simulink model "TwoLinkCartesianNN"  (Simulink 7.6)
settings: Solver=ode45  StartTime=0.0  StopTime=10.0  RelTol=1e-3
libraries: neural x148, roblocks x3, simulink x1
(part 1 of 5)
settings Model: Creator=mahyar  LastModifiedBy=mahyar

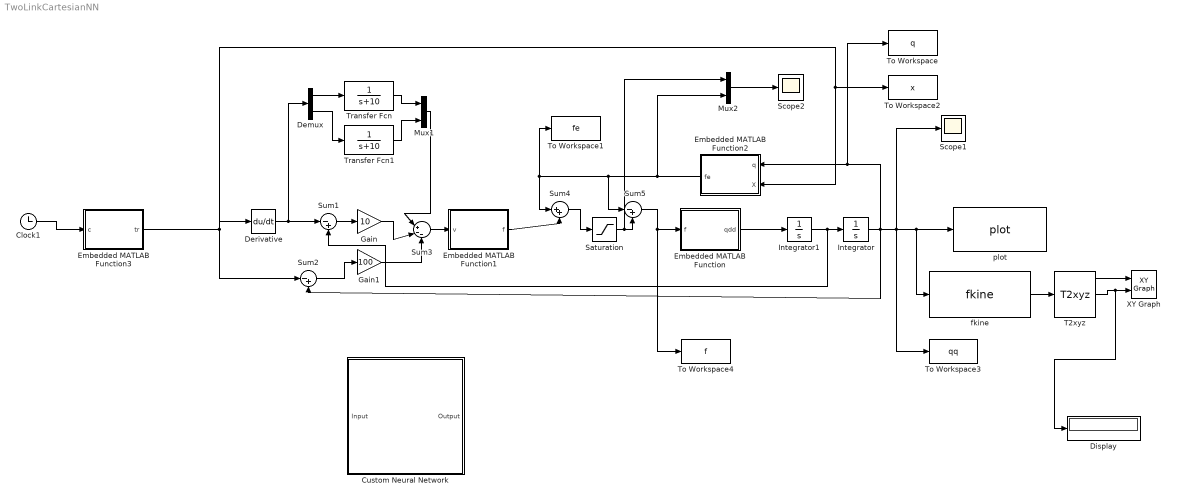
== system TwoLinkCartesianNN ==
  Clock1 : Clock
      settings: Decimation=10
  Custom Neural Network : Subsystem
      mask Description: Custom Neural Network
      mask Display: e = 0.06;c1 = [120 150 230]/255;c2 = ([120 150 230]+0)/383;c3 = ([120 150 230]+128)/383;patch([0 1 1 0],[0 0 1 1],c1);patch([0 1 1 1-e 1-e 0+e],[0 0 1 1-e 0+e 0+e],c2);patch([0 0 1 1-e 0+e 0+e],[0 1 1 1-e 1-e 0+e],c3);plot([0 1 1 0 0],[0 0 1 1 0]);fprintf('NNET');port_label('input',1,' Input');port_label('output',1,'Output ');
  Demux : Demux  Outputs=2
  Derivative : Derivative
  Display : Display
  Embedded MATLAB Function : Stateflow chart  TreatAsAtomicUnit=on
  Embedded MATLAB Function1 : Stateflow chart  TreatAsAtomicUnit=on
  Embedded MATLAB Function2 : Stateflow chart  TreatAsAtomicUnit=on
  Embedded MATLAB Function3 : Stateflow chart  TreatAsAtomicUnit=on
  Gain : Gain  Gain=10
  Gain1 : Gain  Gain=100
  Integrator : Integrator  InitialCondition=[0;0]
  Integrator1 : Integrator  InitialCondition=[0 ;0]
  Mux1 : Mux  Inputs=2
  Mux2 : Mux  Inputs=2
  Saturation : Saturate  UpperLimit=80  LowerLimit=-80
  Scope1 : Scope
      settings: YMin=0  YMax=1.2
  Scope2 : Scope
      settings: TimeRange=10  YMin=-7e+07  YMax=8e+07  SaveName=ScopeData2
  Sum1 : Sum  Inputs=|-+
  Sum2 : Sum  Inputs=|-+
  Sum3 : Sum  Inputs=|+--
  Sum4 : Sum  Inputs=|++
  Sum5 : Sum  Inputs=|-+
  T2xyz : roblocks/T2xyz  SystemSampleTime=-1
  To Workspace : ToWorkspace  VariableName=q  SampleTime=-1  SaveFormat=Structure
  To Workspace1 : ToWorkspace  VariableName=fe  SampleTime=-1  SaveFormat=Structure
  To Workspace2 : ToWorkspace  VariableName=x  SampleTime=-1  SaveFormat=Structure
  To Workspace3 : ToWorkspace  VariableName=qq  SampleTime=-1  SaveFormat=Structure
  To Workspace4 : ToWorkspace  VariableName=f  SampleTime=-1  SaveFormat=Structure
  Transfer Fcn : TransferFcn  Denominator=[1 10]
  Transfer Fcn1 : TransferFcn  Denominator=[1 10]
  XY Graph : simulink/Sinks/XY Graph  SystemSampleTime=-1  xmin=-4  xmax=4  ymin=-4  ymax=4  st=-1
  fkine : roblocks/fkine  SystemSampleTime=-1  robot=r
  plot : roblocks/plot  SystemSampleTime=-1  robot=r
  wires:
  fkine/1 -> T2xyz/1
  Embedded MATLAB Function/1(qdd) -> Integrator1/1
  Integrator/1 -> plot/1, fkine/1, Scope1/1, To Workspace3/1, Sum2/2, Embedded MATLAB Function2/1(q), To Workspace/1
  Integrator1/1 -> Integrator/1, Sum1/2
  Derivative/1 -> Sum1/1, Demux/1
  Sum3/1 -> Embedded MATLAB Function1/1(v)
  Sum1/1 -> Gain/1
  Gain/1 -> Sum3/2
  Sum2/1 -> Gain1/1
  Gain1/1 -> Sum3/3
  Demux/1 -> Transfer Fcn/1
  Demux/2 -> Transfer Fcn1/1
  Transfer Fcn/1 -> Mux1/1
  Transfer Fcn1/1 -> Mux1/2
  Mux1/1 -> Sum3/1
  Embedded MATLAB Function2/1(fe) -> Mux2/2, Sum5/1, Sum4/1, To Workspace1/1
  Mux2/1 -> Scope2/1
  Embedded MATLAB Function1/1(f) -> Sum4/2
  Embedded MATLAB Function3/1(tr) -> Derivative/1, Sum2/1, Embedded MATLAB Function2/2(X), To Workspace2/1
  T2xyz/1 -> XY Graph/1
  T2xyz/2 -> XY Graph/2, Display/1
  Sum5/1 -> Embedded MATLAB Function/1(f), To Workspace4/1
  Sum4/1 -> Saturation/1
  Saturation/1 -> Sum5/2, Mux2/1
  Clock1/1 -> Embedded MATLAB Function3/1(c)

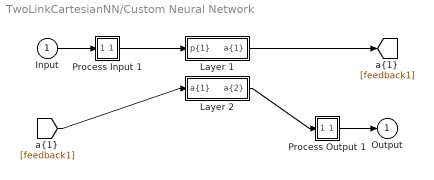
== system TwoLinkCartesianNN/Custom Neural Network ==
  Input : Inport  PortDimensions=131
      mask Display: e = 0.06;c1 = [120 230 180]/255;c2 = ([120 230 180]+0)/(256+128);c3 = ([120 230 180]+128)/(256+128);patch([0 1 1 0],[0 0 1 1],c1);patch([0 1 1 1-e 1-e 0+e],[0 0 1 1-e 0+e 0+e],c2);patch([0 0 1 1-e 0+e 0+e],[0 1 1 1-e 1-e 0+e],c3);plot([0 1 1 0 0],[0 0 1 1 0]);
  Layer 1 : Subsystem
      mask Display: e = 0.06;c1 = [120 150 230]/255;c2 = ([120 150 230]+0)/383;c3 = ([120 150 230]+128)/383;patch([0 1 1 0],[0 0 1 1],c1);patch([0 1 1 1-e 1-e 0+e],[0 0 1 1-e 0+e 0+e],c2);patch([0 0 1 1-e 0+e 0+e],[0 1 1 1-e 1-e 0+e],c3);plot([0 1 1 0 0],[0 0 1 1 0]);
  Layer 2 : Subsystem
      mask Display: e = 0.06;c1 = [120 150 230]/255;c2 = ([120 150 230]+0)/383;c3 = ([120 150 230]+128)/383;patch([0 1 1 0],[0 0 1 1],c1);patch([0 1 1 1-e 1-e 0+e],[0 0 1 1-e 0+e 0+e],c2);patch([0 0 1 1-e 0+e 0+e],[0 1 1 1-e 1-e 0+e],c3);plot([0 1 1 0 0],[0 0 1 1 0]);
  Process Input 1 : Subsystem
      mask Display: e = 0.06;c1 = [120 150 230]/255;c2 = ([120 150 230]+0)/383;c3 = ([120 150 230]+128)/383;patch([0 1 1 0],[0 0 1 1],c1);patch([0 1 1 1-e 1-e 0+e],[0 0 1 1-e 0+e 0+e],c2);patch([0 0 1 1-e 0+e 0+e],[0 1 1 1-e 1-e 0+e],c3);plot([0 1 1 0 0],[0 0 1 1 0]);
  Process Output 1 : Subsystem
      mask Display: e = 0.06;c1 = [120 150 230]/255;c2 = ([120 150 230]+0)/383;c3 = ([120 150 230]+128)/383;patch([0 1 1 0],[0 0 1 1],c1);patch([0 1 1 1-e 1-e 0+e],[0 0 1 1-e 0+e 0+e],c2);patch([0 0 1 1-e 0+e 0+e],[0 1 1 1-e 1-e 0+e],c3);plot([0 1 1 0 0],[0 0 1 1 0]);
  Output : Outport  InitialOutput=[0;0;0;0;0;0;0;0;0;0;0;0;0;0;0;0;0;0;0;0;0;0;0;0;0;0;0;0;0;0;0;0;0;0;0;0;0;0;0;0;0;0;0;0;0;0;0;0;0;0;0;0;0;0;0;0;0;0;0;0;0;0;0;0;0;0;0;0;0;0;0;0;0;0;0;0;0;0;0;0;0;0;0;0;0;0;0;0;0;0;0;0;0;0;0;0;0;0;0;0;0;0;0;0;0;0;0;0;0;0;0;0;0;0;0;0;0;0;0;0;0;0;0;0;0;0;0;0;0;0;0]
      mask Display: e = 0.06;c1 = [120 230 180]/255;c2 = ([120 230 180]+0)/(256+128);c3 = ([120 230 180]+128)/(256+128);patch([0 1 1 0],[0 0 1 1],c1);patch([0 1 1 1-e 1-e 0+e],[0 0 1 1-e 0+e 0+e],c2);patch([0 0 1 1-e 0+e 0+e],[0 1 1 1-e 1-e 0+e],c3);plot([0 1 1 0 0],[0 0 1 1 0]);
  wires:
  Input/1 -> Process Input 1/1(x)
  Process Output 1/1(y) -> Output/1
  Process Input 1/1(p) -> Layer 1/1("p{1}")
  Layer 1/1("a{1}") -> [feedback1]
  [feedback1] -> Layer 2/1("a{1} ")
  Layer 2/1("a{2}") -> Process Output 1/1(a)

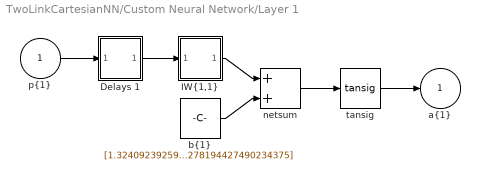
== system TwoLinkCartesianNN/Custom Neural Network/Layer 1 ==
  "p{1}" : Inport  PortDimensions=130
      mask Display: e = 0.06;c1 = [120 230 180]/255;c2 = ([120 230 180]+0)/(256+128);c3 = ([120 230 180]+128)/(256+128);patch([0 1 1 0],[0 0 1 1],c1);patch([0 1 1 1-e 1-e 0+e],[0 0 1 1-e 0+e 0+e],c2);patch([0 0 1 1-e 0+e 0+e],[0 1 1 1-e 1-e 0+e],c3);plot([0 1 1 0 0],[0 0 1 1 0]);
  Delays 1 : Subsystem
      mask Display: e = 0.06;c1 = [120 150 230]/255;c2 = ([120 150 230]+0)/383;c3 = ([120 150 230]+128)/383;patch([0 1 1 0],[0 0 1 1],c1);patch([0 1 1 1-e 1-e 0+e],[0 0 1 1-e 0+e 0+e],c2);patch([0 0 1 1-e 0+e 0+e],[0 1 1 1-e 1-e 0+e],c3);plot([0 1 1 0 0],[0 0 1 1 0]);disp('0');
  "IW{1,1}" : Subsystem
      mask Display: e = 0.06;c1 = [120 150 230]/255;c2 = ([120 150 230]+0)/383;c3 = ([120 150 230]+128)/383;patch([0 1 1 0],[0 0 1 1],c1);patch([0 1 1 1-e 1-e 0+e],[0 0 1 1-e 0+e 0+e],c2);patch([0 0 1 1-e 0+e 0+e],[0 1 1 1-e 1-e 0+e],c3);plot([0 1 1 0 0],[0 0 1 1 0]);disp('W');
  "b{1}" : Constant  Value=[1.3240923925958092421950595962698571383953094482421875;-0.5504773511715745915040542968199588358402252197265625;0.6676637199418795631800094270147383213043212890625;-1.0007797988375102260505400408874265849590301513671875;0.00220576829502830938645185909763313247822225093841552734375;-0.86926988321640508150522919095237739384174346923828125;-0.37316467032025213423906961907050572335720062255859375;-0.99766857705958400526213836201350204646587371826171875;-0.8715553818086945181420333028654567897319793701171875;-1.9230157011015316381730144712491892278194427490234375]
      mask Display: e = 0.06;c1 = [120 150 230]/255;c2 = ([120 150 230]+0)/383;c3 = ([120 150 230]+128)/383;patch([0 1 1 0],[0 0 1 1],c1);patch([0 1 1 1-e 1-e 0+e],[0 0 1 1-e 0+e 0+e],c2);patch([0 0 1 1-e 0+e 0+e],[0 1 1 1-e 1-e 0+e],c3);plot([0 1 1 0 0],[0 0 1 1 0]);disp('b');
  netsum : Sum  Inputs=2  SaturateOnIntegerOverflow=on  InputSameDT=on  OutDataTypeStr=Inherit: Same as first input
      mask Display: e = 0.06;c1 = [120 150 230]/255;c2 = ([120 150 230]+0)/383;c3 = ([120 150 230]+128)/383;patch([0 1 1 0],[0 0 1 1],c1);patch([0 1 1 1-e 1-e 0+e],[0 0 1 1-e 0+e 0+e],c2);patch([0 0 1 1-e 0+e 0+e],[0 1 1 1-e 1-e 0+e],c3);plot([0 1 1 0 0],[0 0 1 1 0]);disp('+');
  tansig : neural/Transfer Functions/tansig  SystemSampleTime=-1
  "a{1}" : Outport  InitialOutput=[0;0;0;0;0;0;0;0;0;0]
      mask Display: e = 0.06;c1 = [120 230 180]/255;c2 = ([120 230 180]+0)/(256+128);c3 = ([120 230 180]+128)/(256+128);patch([0 1 1 0],[0 0 1 1],c1);patch([0 1 1 1-e 1-e 0+e],[0 0 1 1-e 0+e 0+e],c2);patch([0 0 1 1-e 0+e 0+e],[0 1 1 1-e 1-e 0+e],c3);plot([0 1 1 0 0],[0 0 1 1 0]);
  wires:
  "p{1}"/1 -> Delays 1/1("p{1}")
  Delays 1/1("pd{1,1}") -> "IW{1,1}"/1("pd{1,1}")
  "IW{1,1}"/1("iz{1,1}") -> netsum/1
  "b{1}"/1 -> netsum/2
  netsum/1 -> tansig/1
  tansig/1 -> "a{1}"/1

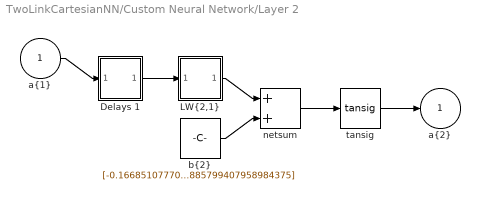
== system TwoLinkCartesianNN/Custom Neural Network/Layer 2 ==
  "a{1} " : Inport  PortDimensions=10
      mask Display: e = 0.06;c1 = [120 230 180]/255;c2 = ([120 230 180]+0)/(256+128);c3 = ([120 230 180]+128)/(256+128);patch([0 1 1 0],[0 0 1 1],c1);patch([0 1 1 1-e 1-e 0+e],[0 0 1 1-e 0+e 0+e],c2);patch([0 0 1 1-e 0+e 0+e],[0 1 1 1-e 1-e 0+e],c3);plot([0 1 1 0 0],[0 0 1 1 0]);
  Delays 1 : Subsystem
      mask Display: e = 0.06;c1 = [120 150 230]/255;c2 = ([120 150 230]+0)/383;c3 = ([120 150 230]+128)/383;patch([0 1 1 0],[0 0 1 1],c1);patch([0 1 1 1-e 1-e 0+e],[0 0 1 1-e 0+e 0+e],c2);patch([0 0 1 1-e 0+e 0+e],[0 1 1 1-e 1-e 0+e],c3);plot([0 1 1 0 0],[0 0 1 1 0]);disp('0');
  "LW{2,1}" : Subsystem
      mask Display: e = 0.06;c1 = [120 150 230]/255;c2 = ([120 150 230]+0)/383;c3 = ([120 150 230]+128)/383;patch([0 1 1 0],[0 0 1 1],c1);patch([0 1 1 1-e 1-e 0+e],[0 0 1 1-e 0+e 0+e],c2);patch([0 0 1 1-e 0+e 0+e],[0 1 1 1-e 1-e 0+e],c3);plot([0 1 1 0 0],[0 0 1 1 0]);disp('W');
  "b{2}" : Constant  Value=[-0.166851077700779837353906032149097882211208343505859375;-0.7843861402824192641247691426542587578296661376953125;-1.21899199102033239938691622228361666202545166015625;0.74462505282958513230795460913213901221752166748046875;-14.41248836651606524128510500304400920867919921875;-0.50346793045477788997033030682359822094440460205078125;-0.08879336411781564575296243901902926154434680938720703125;0.5949153939878153440901087378733791410923004150390625;-0.23842351826200747222372910982812754809856414794921875;0.08428080431664590477236487231493811123073101043701171875;2.475390507348269597542866904404945671558380126953125;-1.515487985379832647225839536986313760280609130859375;-1.4841112529706073086543938188697211444377899169921875;-3.698697968380269873733823260408826172351837158203125;1.3190452876237037660445139408693648874759674072265625;-0.577684328874242591922438805340789258480072021484375;0.37709011321786067849615164959686808288097381591796875;4.10059286012625623385474682436324656009674072265625;-1.32830989378755948138177700457163155078887939453125;-0.640354700549860211822306155227124691009521484375;-0.9377771361900177904402653439319692552089691162109375;-0.332323286094457659434198149028816260397434234619140625;-0.491597104001876006318383360849111340939998626708984375;-0.33628881344515093587688170373439788818359375;-0.89967439422496031653508907766081392765045166015625;-0.6323618525322995953530380575102753937244415283203125;0.68337225464510320538380483412765897810459136962890625;0.2793558622674485736325777907040901482105255126953125;-0.201525497936521802433418315558810718357563018798828125;0.11879681172828326918278207813273184001445770263671875;-0.00629195051082419298804637719513266347348690032958984375;0.315698408201655678073649369252962060272693634033203125;0.2548898739333729235312375749344937503337860107421875;-0.94370324940252425793829615940921939909458160400390625;-0.47721574682566070269018609906197525560855865478515625;-0.41159665142540247106950346278608776628971099853515625;-0.59614215420473015694113883000682108104228973388671875;-0.45437374897230331516340129383024759590625762939453125;0.325243631150170298127477508387528359889984130859375;0.020432118758119656443117406752207898534834384918212890625;-0.0738731793699264616126498594894655980169773101806640625;-0.14508218113239390589797039865516126155853271484375;0.1505264641359329302883196533002774231135845184326171875;-0.06821648328257075288849620164910447783768177032470703125;-0.231870568506500174255080537477624602615833282470703125;0.0967403775629794016044371574025717563927173614501953125;0.57078388551450431886991054852842353284358978271484375;1.045708075089812449931514493073336780071258544921875;1.3787610353289398990028757907566614449024200439453125;0.339027955795436763963834891910664737224578857421875;0.545951479721761501195942400954663753509521484375;0.09048094402358418386622673779129399918019771575927734375;-0.812040329819399442357052976149134337902069091796875;-0.0553867262122519632416839385768980719149112701416015625;-0.66903156004904129616761565557681024074554443359375;-0.1815240657789118638998360211189719848334789276123046875;-0.6668235261192074769809323697700165212154388427734375;-0.35750263343022792295045064747682772576808929443359375;0.0827722526877872066819463725551031529903411865234375;0.251478809341716014191803196808905340731143951416015625;4.52587391069360034379087665001861751079559326171875;-0.05396634953846461690840641267641331069171428680419921875;0.01061590559154333701652461741105071268975734710693359375;0.50455607095879084766920641413889825344085693359375;-0.0661537821694408723072200473325210623443126678466796875;0.0205873683818567389247622401171611272729933261871337890625;-0.1439892528579400643451435826136730611324310302734375;0.28208297214947375408655716455541551113128662109375;0.11076787990505952696818070535300648771226406097412109375;-0.467520686277630714844377735062153078615665435791015625;0.0564319078922222161498467585261096246540546417236328125 ...(+3348 chars)]
      mask Display: e = 0.06;c1 = [120 150 230]/255;c2 = ([120 150 230]+0)/383;c3 = ([120 150 230]+128)/383;patch([0 1 1 0],[0 0 1 1],c1);patch([0 1 1 1-e 1-e 0+e],[0 0 1 1-e 0+e 0+e],c2);patch([0 0 1 1-e 0+e 0+e],[0 1 1 1-e 1-e 0+e],c3);plot([0 1 1 0 0],[0 0 1 1 0]);disp('b');
  netsum : Sum  Inputs=2  SaturateOnIntegerOverflow=on  InputSameDT=on  OutDataTypeStr=Inherit: Same as first input
      mask Display: e = 0.06;c1 = [120 150 230]/255;c2 = ([120 150 230]+0)/383;c3 = ([120 150 230]+128)/383;patch([0 1 1 0],[0 0 1 1],c1);patch([0 1 1 1-e 1-e 0+e],[0 0 1 1-e 0+e 0+e],c2);patch([0 0 1 1-e 0+e 0+e],[0 1 1 1-e 1-e 0+e],c3);plot([0 1 1 0 0],[0 0 1 1 0]);disp('+');
  tansig : neural/Transfer Functions/tansig  SystemSampleTime=-1
  "a{2}" : Outport  InitialOutput=[0;0;0;0;0;0;0;0;0;0;0;0;0;0;0;0;0;0;0;0;0;0;0;0;0;0;0;0;0;0;0;0;0;0;0;0;0;0;0;0;0;0;0;0;0;0;0;0;0;0;0;0;0;0;0;0;0;0;0;0;0;0;0;0;0;0;0;0;0;0;0;0;0;0;0;0;0;0;0;0;0;0;0;0;0;0;0;0;0;0;0;0;0;0;0;0;0;0;0;0;0;0;0;0;0;0;0;0;0;0;0;0;0;0;0;0;0;0;0;0;0;0;0;0;0;0;0;0;0;0;0]
      mask Display: e = 0.06;c1 = [120 230 180]/255;c2 = ([120 230 180]+0)/(256+128);c3 = ([120 230 180]+128)/(256+128);patch([0 1 1 0],[0 0 1 1],c1);patch([0 1 1 1-e 1-e 0+e],[0 0 1 1-e 0+e 0+e],c2);patch([0 0 1 1-e 0+e 0+e],[0 1 1 1-e 1-e 0+e],c3);plot([0 1 1 0 0],[0 0 1 1 0]);
  wires:
  "a{1} "/1 -> Delays 1/1("p{2}")
  Delays 1/1("pd{2,1}") -> "LW{2,1}"/1("ad{2,1}")
  "LW{2,1}"/1("lz{2,1}") -> netsum/1
  "b{2}"/1 -> netsum/2
  netsum/1 -> tansig/1
  tansig/1 -> "a{2}"/1

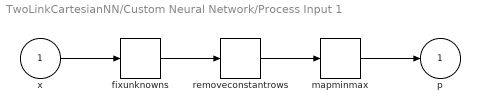
== system TwoLinkCartesianNN/Custom Neural Network/Process Input 1 ==
  x : Inport  PortDimensions=131
      mask Display: e = 0.06;c1 = [120 230 180]/255;c2 = ([120 230 180]+0)/(256+128);c3 = ([120 230 180]+128)/(256+128);patch([0 1 1 0],[0 0 1 1],c1);patch([0 1 1 1-e 1-e 0+e],[0 0 1 1-e 0+e 0+e],c2);patch([0 0 1 1-e 0+e 0+e],[0 1 1 1-e 1-e 0+e],c3);plot([0 1 1 0 0],[0 0 1 1 0]);
  fixunknowns : neural/Processing Functions/fixunknowns  SystemSampleTime=-1  inputSize=131  indices=[1 2 3 4 5 6 7 8 9 10 11 12 13 14 15 16 17 18 19 20 21 22 23 24 25 26 27 28 29 30 31 32 33 34 35 36 37 38 39 40 41 42 43 44 45 46 47 48 49 50 51 52 53 54 55 56 57 58 59 60 61 62 63 64 65 66 67 68 69 70 71 72 73 74 75 76 77 78 79 80 81 82 83 84 85 86 87 88 89 90 91 92 93 94 95 96 97 98 99 100 101 102 103 104 105 106 107 108 109 110 111 112 113 114 115 116 117 118 119 120 121 122 123 124 125 126 127 128 129 130 131]
  mapminmax : neural/Processing Functions/mapminmax  SystemSampleTime=-1  xmin=[0;0;0;0;0;0;0;0;0;0;0;0;0;0;0;0;0;0;0;0;0;0;0;0;0;0;0;0;0;0;0;0;0;0;0;0;0;0;0;0;0;0;0;0;0;0;0;0;0;0;0;0;0;0;0;0;0;0;0;0;0;0;0;0;0;0;0;0;0;0;0;0;3.39127133697992125941339678186e-14;1.94155593837782758925184781959e-13;3.54398474305817057411433895115e-13;5.14641354773887706608195592496e-13;8.35127115710133614268638535189e-13;1.47609863758305467089616051929e-12;2.75804168133061354742935714575e-12;5.32192776883259754581479408544e-12;1.04496999438640321394489766045e-11;2.07052442940367709453448439864e-11;4.12163329948217238004723203404e-11;8.22385103981495304840702394091e-11;1.64282865211836786518729156413e-10;3.28371574867337765860322736756e-10;6.56548994290845593632612882786e-10;1.31290383358788472553360511622e-09;2.62561351398205710155639048685e-09;5.25103288197077871607547111966e-09;1.05018716467497244319239966333e-08;2.10035492915136274652237297587e-08;4.20069050418654633946216733417e-08;8.40136183858650958859338596547e-08;1.68027052447046628446737127904e-07;3.36053950062127196587373305359e-07;6.72107863263064430166737403538e-07;1.34421616154729239181009163573e-06;2.68843464563915471185690311828e-06;5.37687916386845021879435993495e-06;1.07537984001248827033072469339e-05;2.15077576687536199326333807846e-05;4.30161593658708241898550039828e-05;8.6034895202718170820720133829e-05;0.000172080095072320640985780171306;0.00034420139499983192204329851549;0.000688567494861905748590458209435;0.00137779288890775087131346232638;0.00275821001284331027147977977165;0.00552685813998672961777636203351;0.0110949992805678375462630214088;0.0223513934671833273959418164623;0.0453187697715917506280369764227;0.0928695870897397468546330401296;0.192893077264244983126673105289;0.401559002740551396204438105997;0.550000000000000044408920985006;0.550000000000000044408920985006;0.550000000000000044408920985006;0.550000000000000044408920985006;0.550000000000000044408920985006;0.550000000000000044408920985006;0.550000000000000044408920985006;0.550000000000000044408920985006;0.550000000000000044408920985006;0.550000000000000044408920985006;0.550000000000000044408920985006;0.550000000000000044408920985006;0.550000000000000044408920985006;0.550000000000000044408920985006]  xmax=[6.68564073621395946207252206599e-10;2.40683066503702594401350610322e-08;6.42490074750161794335371646947e-07;1.62701752956502980549790410292e-05;0.000407798010910180759591714405587;0.0102001724267335759643859915968;0.0590865656757802448773020387307;0.05908656567578192408962678428;0.248304885285112464377021979089;0.448669105191036199364873482409;0.5890397005128985563615628962;0.637646357032778721141141886619;0.603709527915894494931592362263;0.557523021740516044886248891999;0.536800209363013203223147229437;0.540689393306072352274327386112;0.55058918842240767155260527943;0.552055136888254360805206033547;0.550032803944412118646312137571;0.549750172599031472486785787623;0.550009364327472938249741218897;0.550029657512358438609112454287;0.549997287887633579117618864984;0.549996564654723352205678565952;0.550000510600512027004072024283;0.550000387452318162395670242404;0.549999917700721319135936937528;0.549999957619495050131774860347;0.550000012194730936165854018327;0.550000004465412195564510966506;0.549999998289805169804367324105;0.549999999552185592222031118581;0.550000000230323027317069772835;0.550000000041772296732744962355;0.549999999969969621815835125744;0.549999999996559352233305162372;0.550000000003808553472595122003;0.550000000000212208028926852421;0.549999999999528976779572531086;0.549999999999999600319711134944;0.550000000000056887827781793021;0.549999999999997046806754497084;0.549999999999993383070773234067;0.550000000000000821565038222616;0.550000000000000821565038222616;0.549999999999999933386618522491;0.549999999999999933386618522491;0.550000000000000155431223447522;0.550000000000000155431223447522;0.550000000000000044408920985006;0.550000000000000044408920985006;0.550000000000000044408920985006;0.550000000000000044408920985006;0.550000000000000044408920985006;0.550000000000000044408920985006;0.550000000000000044408920985006;0.550000000000000044408920985006;0.550000000000000044408920985006;0.550000000000000044408920985006;0.550000000000000044408920985006;0.550000000000000044408920985006;0.550000000000000044408920985006;0.550000000000000044408920985006;0.550000000000000044408920985006;0.550000000000000044408920985006;0.550000000000000044408920985006;0.550000000000000044408920985006;0.550000000000000044408920985006;0.550000000000000044408920985006;0.550000000000000044408920985006;0.550000000000000044408920985006;0.550000000000000044408920985006;0.550000000000000044408920985006;0.550000000000000044408920985006;0.550000000000000044408920985006;0.550000000000000044408920985006;0.550000000000000044408920985006;0.550000000000000044408920985006;0.550000000000000044408920985006;0.550000000000000044408920985006;0.550000000000000044408920985006;0.550000000000000044408920985006;0.550000000000000044408920985006;0.550000000000000044408920985006;0.550000000000000044408920985006;0.550000000000000044408920985006;0.550000000000000044408920985006;0.550000000000000044408920985006;0.550000000000000044408920985006;0.550000000000000044408920985006;0.550000000000000044408920985006;0.550000000000000044408920985006;0.550000000000000044408920985006;0.550000000000000044408920985006;0.550000000000000044408920985006;0.550000000000000044408920985006;0.550000000000000044408920985006;0.550000000000000044408920985006;0.550000000000000044408920985006;0.550000000000000044408920985006;0.550000000000000044408920985006;0.550000000000000044408920985006;0.550000000000000044408920985006;0.550000000000000044408920985006;0.550000000000000044408920985006;0.550000000000000044408920985006;0.550000000000000044408920985006;0.550000000000000044408920985006;0.550000000000000044408920985006;0.550000000000000044408920985006;0.550000000000000044408920985006;0.550000000000000044408920985006;0.550000000000000044408920985006;0.550000000000000044408920985006;0.550000000000000044408920985006;0.550000000000000044408920985006;0.785743985268398059673700117855;1.10432497606786705901527056994;1.20164413042005158160918654175;1.12195081313582667448258689546;1.01691014230244780591760900279;0.969569261404452320540769960644;0.978680394311837176246626768261;1.00093087950283621267999478732;1.00483647144235255233013504039;1.00015124969759061634988484002;0.999408144611358295605896273628;1.00001331279962646370051970734;1.00007073431991133638518931548;1.00000940511901337259814681602]  ymin=-1  ymax=1
  removeconstantrows : neural/Processing Functions/removeconstantrows  SystemSampleTime=-1  inputSize=131  keep=[2 3 4 5 6 7 8 9 10 11 12 13 14 15 16 17 18 19 20 21 22 23 24 25 26 27 28 29 30 31 32 33 34 35 36 37 38 39 40 41 42 43 44 45 46 47 48 49 50 51 52 53 54 55 56 57 58 59 60 61 62 63 64 65 66 67 68 69 70 71 72 73 74 75 76 77 78 79 80 81 82 83 84 85 86 87 88 89 90 91 92 93 94 95 96 97 98 99 100 101 102 103 104 105 106 107 108 109 110 111 112 113 114 115 116 117 118 119 120 121 122 123 124 125 126 127 128 129 130 131]
  p : Outport  PortDimensions=130
      mask Display: e = 0.06;c1 = [120 230 180]/255;c2 = ([120 230 180]+0)/(256+128);c3 = ([120 230 180]+128)/(256+128);patch([0 1 1 0],[0 0 1 1],c1);patch([0 1 1 1-e 1-e 0+e],[0 0 1 1-e 0+e 0+e],c2);patch([0 0 1 1-e 0+e 0+e],[0 1 1 1-e 1-e 0+e],c3);plot([0 1 1 0 0],[0 0 1 1 0]);
  wires:
  x/1 -> fixunknowns/1
  fixunknowns/1 -> removeconstantrows/1
  removeconstantrows/1 -> mapminmax/1
  mapminmax/1 -> p/1

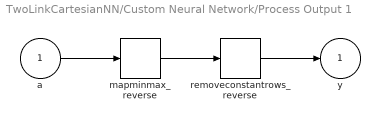
== system TwoLinkCartesianNN/Custom Neural Network/Process Output 1 ==
  a : Inport  PortDimensions=131
      mask Display: e = 0.06;c1 = [120 230 180]/255;c2 = ([120 230 180]+0)/(256+128);c3 = ([120 230 180]+128)/(256+128);patch([0 1 1 0],[0 0 1 1],c1);patch([0 1 1 1-e 1-e 0+e],[0 0 1 1-e 0+e 0+e],c2);patch([0 0 1 1-e 0+e 0+e],[0 1 1 1-e 1-e 0+e],c3);plot([0 1 1 0 0],[0 0 1 1 0]);
  mapminmax_reverse : neural/Processing Functions/mapminmax_reverse  SystemSampleTime=-1  xmin=[0;0;0;0;0;0;0;0;0;0;-7.69111613108554337259192834608;-11.3245418689005283852111460874;0;0;0;0;0;0;0;0;0;0;0;0;0;0;0;0;0;0;0;0;0;0;0;0;0;0;0;0;0;0;0;0;0;0;0;0;0;0;0;0;0;0;0;0;0;0;0;0;0;0;0;0;0;0;0;0;0;0;0;0;0;19.6000000000000014210854715202;19.6000000000000014210854715202;19.6000000000000014210854715202;19.6000000000000014210854715202;19.6000000000000014210854715202;19.6000000000000014210854715202;19.6000000000000014210854715202;19.6000000000000014210854715202;19.6000000000000014210854715202;19.6000000000000014210854715202;19.6000000000000014210854715202;19.6000000000000014210854715202;19.6000000000000014210854715202;19.6000000000000014210854715202;19.6000000000000014210854715202;19.6000000000000014210854715202;19.6000000000000014210854715202;19.6000000000000014210854715202;19.6000000000000014210854715202;19.6000000000000014210854715202;19.6000000000000014210854715202;19.6000000000000014210854715202;19.6000000000000014210854715202;19.6000000000000014210854715202;19.6000000000000014210854715202;19.6000000000000014210854715202;19.6000000000000014210854715202;19.6000000000000014210854715202;19.6000000000000014210854715202;19.6000000000000014210854715202;19.6000000000000014210854715202;19.6000000000000014210854715202;19.6000000000000014210854715202;19.6000000000000014210854715202;19.6000000000000014210854715202;19.6000000000000014210854715202;19.6000000000000014210854715202;19.6000000000000014210854715202;19.6000000000000014210854715202;19.6000000000000014210854715202;19.6000000000000014210854715202;19.6000000000000014210854715202;15.6123115434016597191657638177;-6.61632391140367559501100913621;-31.896922571551080238805297995;-34.9612760390082257799804210663;-19.0761881515679263543461274821;-1.22771317830014758953893760918;5.81354441599272675489373796154;4.43975289352101398776540008839;0.382749454541473133062368106039;-0.961294993809252651395524935651;-0.311845260014274039406245719874;0.139398903401628249110189017301;0.0302112900056430606909874114763;-0.0184377955225226743130040318874;-0.00266340785900803529023805893416;0.00256580766025863620319324986951]  xmax=[80;80;80;80;80;80;80;80;79.9999999999991473487170878798;21.2206086643731168805970810354;0;0;1.94581048423367519717430695891;18.3556612574125281867054582108;24.6424854909974868633071309887;23.4740549159158256031787459506;19.9425280316086883658499573357;18.7726606628105372465142863803;19.3506825137917992663005861687;19.7211959201175872635758423712;19.6236316083733619564100081334;19.584109953373889823069475824;19.5979948714493019679139251821;19.6020250453732138851137278834;19.6001340388753710897162818583;19.5997484057829289838537079049;19.5999972383766554173689655727;19.6000305175040701044508750783;19.5999987057584235117246862501;19.5999963852244114548284414923;19.6000003490173710929411754478;19.6000004177293298823769873707;19.5999999355908265386005950859;19.5999999530105846190508600557;19.6000000102810147950549435336;19.600000005123821011920881574;19.5999999984856820844925096026;19.5999999994622768895169429015;19.600000000211483808243428939;19.6000000000536260813532862812;19.5999999999716081333644979168;19.5999999999950560436445812229;19.6000000000036855851703876397;19.6000000000003993250174971763;19.5999999999995218047388334526;19.5999999999999694466623623157;19.6000000000000511590769747272;19.6000000000000049737991503207;19.5999999999999587885213259142;19.5999999999999978683717927197;19.5999999999999978683717927197;19.6000000000000014210854715202;19.6000000000000014210854715202;19.6000000000000014210854715202;19.6000000000000014210854715202;19.6000000000000014210854715202;19.6000000000000014210854715202;19.6000000000000014210854715202;19.6000000000000014210854715202;19.6000000000000014210854715202;19.6000000000000014210854715202;19.6000000000000014210854715202;19.6000000000000014210854715202;19.6000000000000014210854715202;19.6000000000000014210854715202;19.6000000000000014210854715202;19.6000000000000014210854715202;19.6000000000000014210854715202;19.6000000000000014210854715202;19.6000000000000014210854715202;19.6000000000000014210854715202;19.6000000000000014210854715202;19.6000000000000014210854715202;80;44.2744990366817461335813277401;44.2744990366529478365009708796;44.27449903662415664484797162;44.274499036566552945259900298;44.2744990364513739677931880578;44.2744990362210302237144787796;44.2744990357603214192749874201;44.274499034838903810396004701;44.274499032996104119774827268;44.2744990293104763168230419978;44.2744990219392065000647562556;44.2744990071966739719755423721;44.2744989777116231266518298071;44.2744989187414859088676166721;44.274498800801247000435978407;44.274498564920754972717986675;44.2744980931597709172820032109;44.2744971496377957009826786816;44.2744952625938665846661024261;44.2744914885060794063065259252;44.2744839403307679503996041603;44.2744688439810758495696063619;44.2744386512855285786827153061;44.2743782659098528142749273684;44.2742574952199774429573153611;44.2740159540861384357413044199;44.2735328728022921040974324569;44.2725667141698266959792817943;44.2706344126458262167034263257;44.2667698725628468991999397986;44.2590410442650821210008871276;44.2435843952092682229704223573;44.212675127790141971217963146;44.1508727199903674431880062912;44.0273324466451256853360973764;43.7805103410483340553582820576;43.287902059208214211594167864;42.3068463470526268110916134901;40.3615124430830860546848271042;36.5389807076262300711277930532;29.1739322215615572986280312762;19.6000000000000014210854715202;19.6000000000000014210854715202;19.6000000000000014210854715202;19.6000000000000014210854715202;19.6000000000000014210854715202;19.6000000000000014210854715202;19.6000000000000014210854715202;19.6000000000000014210854715202;19.6000000000000014210854715202;19.6000000000000014210854715202;19.6000000000000014210854715202;19.6000000000000014210854715202;19.6000000000000014210854715202;19.6000000000000014210854715202;19.6000000000000014210854715202;19.6000000000000014210854715202]  ymin=-1  ymax=1
  removeconstantrows_reverse : neural/Processing Functions/removeconstantrows_reverse  SystemSampleTime=-1  inputSize=131  constants=zeros(0,1)  rearrange=[1 2 3 4 5 6 7 8 9 10 11 12 13 14 15 16 17 18 19 20 21 22 23 24 25 26 27 28 29 30 31 32 33 34 35 36 37 38 39 40 41 42 43 44 45 46 47 48 49 50 51 52 53 54 55 56 57 58 59 60 61 62 63 64 65 66 67 68 69 70 71 72 73 74 75 76 77 78 79 80 81 82 83 84 85 86 87 88 89 90 91 92 93 94 95 96 97 98 99 100 101 102 103 104 105 106 107 108 109 110 111 112 113 114 115 116 117 118 119 120 121 122 123 124 125 126 127 128 129 130 131]
  y : Outport  PortDimensions=131
      mask Display: e = 0.06;c1 = [120 230 180]/255;c2 = ([120 230 180]+0)/(256+128);c3 = ([120 230 180]+128)/(256+128);patch([0 1 1 0],[0 0 1 1],c1);patch([0 1 1 1-e 1-e 0+e],[0 0 1 1-e 0+e 0+e],c2);patch([0 0 1 1-e 0+e 0+e],[0 1 1 1-e 1-e 0+e],c3);plot([0 1 1 0 0],[0 0 1 1 0]);
  wires:
  a/1 -> mapminmax_reverse/1
  mapminmax_reverse/1 -> removeconstantrows_reverse/1
  removeconstantrows_reverse/1 -> y/1

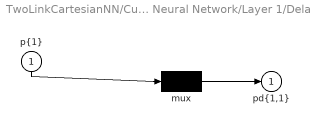
== system TwoLinkCartesianNN/Custom Neural Network/Layer 1/Delays 1 ==
  "p{1}" : Inport  PortDimensions=130
      mask Display: e = 0.06;c1 = [120 230 180]/255;c2 = ([120 230 180]+0)/(256+128);c3 = ([120 230 180]+128)/(256+128);patch([0 1 1 0],[0 0 1 1],c1);patch([0 1 1 1-e 1-e 0+e],[0 0 1 1-e 0+e 0+e],c2);patch([0 0 1 1-e 0+e 0+e],[0 1 1 1-e 1-e 0+e],c3);plot([0 1 1 0 0],[0 0 1 1 0]);
  mux : Mux  Inputs=1
      mask Display: e = 0.06;c1 = [120 150 230]/255;c2 = ([120 150 230]+0)/383;c3 = ([120 150 230]+128)/383;patch([0 1 1 0],[0 0 1 1],c1);patch([0 1 1 1-e 1-e 0+e],[0 0 1 1-e 0+e 0+e],c2);patch([0 0 1 1-e 0+e 0+e],[0 1 1 1-e 1-e 0+e],c3);plot([0 1 1 0 0],[0 0 1 1 0]);disp('Mux')
  "pd{1,1}" : Outport
      mask Display: e = 0.06;c1 = [120 230 180]/255;c2 = ([120 230 180]+0)/(256+128);c3 = ([120 230 180]+128)/(256+128);patch([0 1 1 0],[0 0 1 1],c1);patch([0 1 1 1-e 1-e 0+e],[0 0 1 1-e 0+e 0+e],c2);patch([0 0 1 1-e 0+e 0+e],[0 1 1 1-e 1-e 0+e],c3);plot([0 1 1 0 0],[0 0 1 1 0]);
  wires:
  "p{1}"/1 -> mux/1
  mux/1 -> "pd{1,1}"/1
